simulink model "C_h_enrutm"  (R2020b)
settings: Solver=VariableStepAuto  StartTime=0.0  StopTime=1.5  RelTol=1e-3
settings Model: Creator=retou  LastModifiedBy=retou

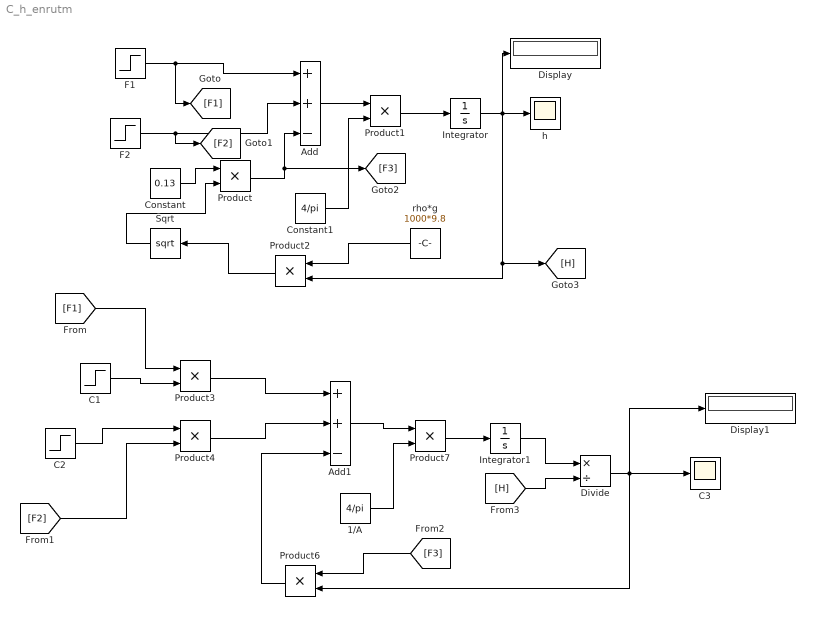
== system C_h_enrutm ==
  1/A : Constant  Value=4/pi
  Add : Sum  Inputs=++-
  Add1 : Sum  Inputs=++-
  C1 : Step  Time=0  Before=10  After=10*1.2  SampleTime=0
  C2 : Step  Time=0  Before=3  After=3  SampleTime=0
  C3 : Scope
  Constant : Constant  Value=0.13
  Constant1 : Constant  Value=4/pi
  Display : Display
  Display1 : Display
  Divide : Product  Inputs=*/
  F1 : Step  Time=0  Before=6  After=6  SampleTime=0
  F2 : Step  Time=0  Before=12  After=12  SampleTime=0
  Integrator : Integrator  InitialCondition=1.956
  Integrator1 : Integrator  InitialCondition=5.33*1.956
  Product{,1..4,6..7} (7 alike) : Product
  Sqrt : Sqrt  SaturateOnIntegerOverflow=on
  h : Scope
  rho*g : Constant  Value=1000*9.8
  wires:
  F1/1 -> [F1], Add/1
  F2/1 -> [F2], Add/2
  Constant/1 -> Product/1
  Sqrt/1 -> Product/2
  Product/1 -> [F3], Add/3
  Add/1 -> Product1/1
  Constant1/1 -> Product1/2
  Product1/1 -> Integrator/1
  Integrator/1 -> Product2/2, [H], Display/1, h/1
  Product2/1 -> Sqrt/1
  rho*g/1 -> Product2/1
  C2/1 -> Product4/1
  [F2] -> Product4/2
  [F1] -> Product3/1
  C1/1 -> Product3/2
  Product3/1 -> Add1/1
  Product4/1 -> Add1/2
  Product6/1 -> Add1/3
  Add1/1 -> Product7/1
  1/A/1 -> Product7/2
  Product7/1 -> Integrator1/1
  Integrator1/1 -> Divide/1
  Divide/1 -> C3/1, Product6/2, Display1/1
  [F3] -> Product6/1
  [H] -> Divide/2
